simulink model "FDM"  (R2023b)
settings: Solver=VariableStepAuto  StartTime=0.0  StopTime=10.0  RelTol=1e-3
settings Model: Creator=maruv  LastModifiedBy=maruv

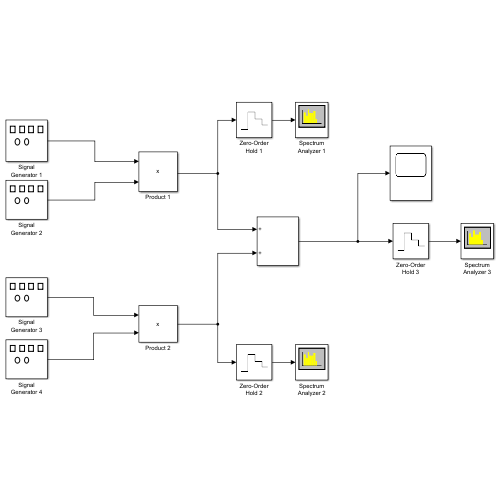
[thumbnail: Simulink's stored preview of the top-level diagram]
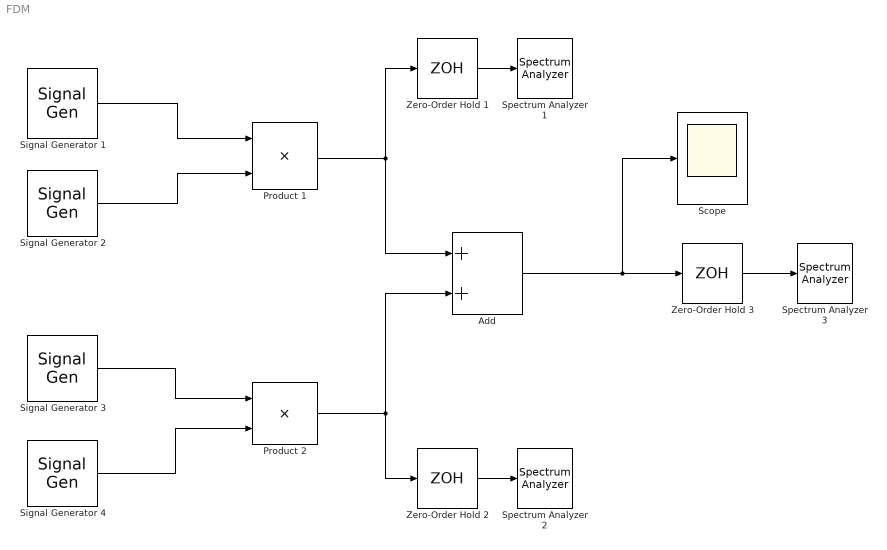
== system FDM ==
  Add : Sum
  Product 1 : Product
  Product 2 : Product
  Scope : Scope
  Signal Generator 1 : SignalGenerator  Frequency=100
  Signal Generator 2 : SignalGenerator  Frequency=1000
  Signal Generator 3 : SignalGenerator  Frequency=200  VectorParams1D=off
  Signal Generator 4 : SignalGenerator  Frequency=2000
  Spectrum Analyzer 1 : SpectrumAnalyzer  WindowPosition=[770.000000,2.000000,766.000000,401.000000,]  ScopeFrameLocation=window  Span=40000  StartFrequency=-20000  StopFrequency=20000  YLimits=[-258.5032597,48.6768078]
  Spectrum Analyzer 2 : SpectrumAnalyzer  WindowPosition=[770.000000,434.000000,766.000000,401.000000,]  ScopeFrameLocation=window  YLimits=[-254.67494363,48.25143797]
  Spectrum Analyzer 3 : SpectrumAnalyzer  WindowPosition=[2.000000,2.000000,766.000000,833.000000,]  ScopeFrameLocation=window  YLimits=[-253.33413665,48.1024608]
  Zero-Order Hold 1 : ZeroOrderHold  SampleTime=-1
  Zero-Order Hold 2 : ZeroOrderHold  SampleTime=-1
  Zero-Order Hold 3 : ZeroOrderHold  SampleTime=1/40000
  wires:
  Signal Generator 3/1 -> Product 2/1
  Signal Generator 4/1 -> Product 2/2
  Signal Generator 1/1 -> Product 1/1
  Signal Generator 2/1 -> Product 1/2
  Product 1/1 -> Zero-Order Hold 1/1, Add/1
  Product 2/1 -> Add/2, Zero-Order Hold 2/1
  Zero-Order Hold 1/1 -> Spectrum Analyzer 1/1
  Zero-Order Hold 2/1 -> Spectrum Analyzer 2/1
  Add/1 -> Scope/1, Zero-Order Hold 3/1
  Zero-Order Hold 3/1 -> Spectrum Analyzer 3/1
